simulink model "cb_pcidda_test"  (Simulink 4.00)
settings: Solver=FixedStepDiscrete  SolverMode=MultiTasking  StartTime=0.0  StopTime=1  RelTol=1e-3
libraries: cb_pcidda x7
CloseFcn:
  | rtwprivate ssgensfun ModelCloseRequest cb_pcidda_test
settings Model: Creator=dozio  LastModifiedBy=root  SimulationMode=external  RTWSystemTargetFile=grt_rtai.tlc  RTWOptions="-aBasePriority=30 -aExtMode=1 -aForceParamTrailComments=0 -aInlineInvariantSignals=0 -aInlineParameters=0 -aLocalBlockOutputs=1 -aLogVarNameModifier=\"rt_\" -aMatFileLogging=0 -aRTWVerbose=1 -aRollThreshold=5 -aShowEliminatedStatements=1 -aTaskStackSize=16384"  RTWTemplateMakefile=grt_rtai.tmf  BlockReductionOpt=off

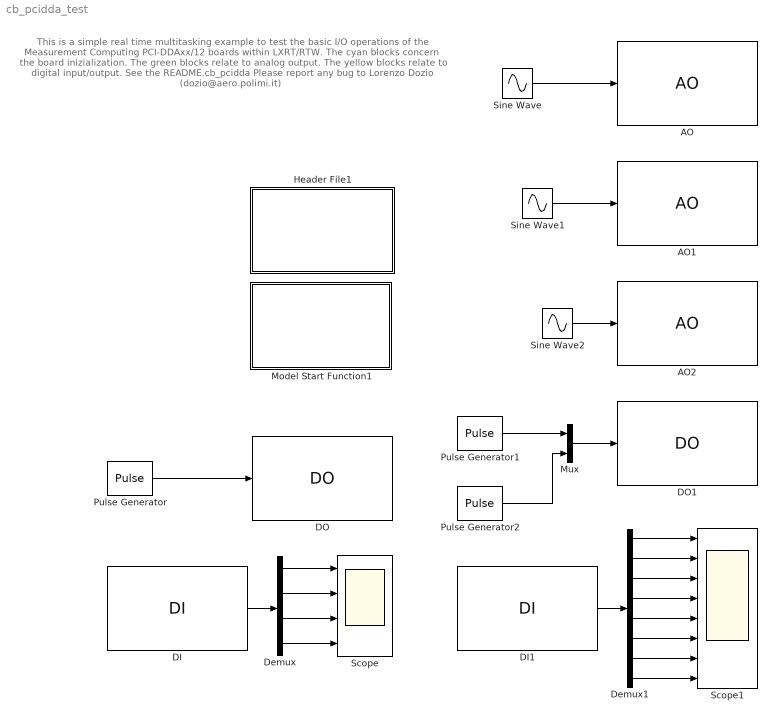
== system cb_pcidda_test ==
  note: This is a simple real time multitasking example to test
      | the basic I/O operations of the Measurement Computing
      | PCI-DDAxx/12 boards within LXRT/RTW.
      | The cyan blocks concern the board inizialization.
      | The green blocks relate to analog output.
      | The yellow blocks relate to digital input/output.
      | See the README.cb_pcidda
      |
      | Please report any bug to Lorenzo Dozio
      | (dozio@aero.polimi.it)
  AO : cb_pcidda/AO  chan=DAC0  pol=bipolar  vfs=10 V  dt=0.0001
  AO1 : cb_pcidda/AO  chan=DAC1  pol=unipolar  vfs=5 V  dt=0.0002
  AO2 : cb_pcidda/AO  chan=DAC2  pol=bipolar  vfs=10 V  dt=0.0004
  DI : cb_pcidda/DI  number=0  port=C_up  nchan=4  dt=0.0005
  DI1 : cb_pcidda/DI  number=1  port=A  nchan=8  dt=0.0005
  DO : cb_pcidda/DO  number=0  port=C_low  nchan=1  threshold=1  dt=0.0005
  DO1 : cb_pcidda/DO  number=1  port=B  nchan=2  threshold=1  dt=0.0005
  Demux : Demux  Outputs=4  BusSelectionMode=off
  Demux1 : Demux  Outputs=8  BusSelectionMode=off
  Header File1 : Subsystem  Tag=line1 line2
      settings: CopyFcn=cccopyfcn(gcb)  OpenFcn=ccopenfcn('Header File')  RTWFcnNameOpts=Auto  RTWFileNameOpts=Auto
      mask Type: Header File
      mask Description: Add code to model .h file
      mask Help: This header file block contains text fields to insert custom user code at the top and bottom of model.h file.
      mask Display: disp('Measurement Computing\nPCI-DDAxx/12\n\nHeader Files');
  Model Start Function1 : Subsystem
      settings: CopyFcn=cccopyfcn(gcb)  OpenFcn=ccopenfcn('Model Start Function')  RTWFcnNameOpts=Auto  RTWFileNameOpts=Auto
      mask Type: Model Start Function
      mask Description: Add code to Model Start function
      mask Help: This block contains text fields to insert custom user code sections at the declarations, execution and exit sections of the model start function.
      mask Display: disp('Measurement Computing\nPCI-DDAxx/12\n\nReset Digital I/O');
  Mux : Mux  Inputs=2
  Pulse Generator : DiscretePulseGenerator  Amplitude=2  Period=50  PulseWidth=25  PhaseDelay=0  SampleTime=0.0005
  Pulse Generator1 : DiscretePulseGenerator  Amplitude=2  Period=50  PulseWidth=25  PhaseDelay=0  SampleTime=0.0005
  Pulse Generator2 : DiscretePulseGenerator  Amplitude=2  Period=50  PulseWidth=25  PhaseDelay=0  SampleTime=0.0005
  Scope : Scope  NumInputPorts=4
      settings: TimeRange=0.1  YMin=0~0~0~0  YMax=1~1~1~1  SaveToWorkspace=off  LimitDataPoints=on  MaxDataPoints=5000
  Scope1 : Scope  NumInputPorts=8
      settings: TimeRange=0.1  YMin=0~0~0~0~0~0~0~0  YMax=1~1~1~1~1~1~1~1  SaveToWorkspace=off  SaveName=ScopeData  LimitDataPoints=on  MaxDataPoints=5000
  Sine Wave : Sin  Amplitude=5  Frequency=2*pi*50  Phase=0  SampleTime=0.0001
  Sine Wave1 : Sin  Amplitude=2.5  Frequency=2*pi*10  Phase=0  SampleTime=0.0002
  Sine Wave2 : Sin  Amplitude=2  Frequency=2*pi*50  Phase=0  SampleTime=0.0004
  wires:
  Sine Wave/1 -> AO/1
  Sine Wave1/1 -> AO1/1
  Sine Wave2/1 -> AO2/1
  Pulse Generator/1 -> DO/1
  DI/1 -> Demux/1
  Demux/1 -> Scope/1
  Demux/2 -> Scope/2
  Demux/3 -> Scope/3
  Demux/4 -> Scope/4
  Pulse Generator1/1 -> Mux/1
  Pulse Generator2/1 -> Mux/2
  Mux/1 -> DO1/1
  DI1/1 -> Demux1/1
  Demux1/1 -> Scope1/1
  Demux1/2 -> Scope1/2
  Demux1/4 -> Scope1/4
  Demux1/3 -> Scope1/3
  Demux1/5 -> Scope1/5
  Demux1/6 -> Scope1/6
  Demux1/7 -> Scope1/7
  Demux1/8 -> Scope1/8

== system cb_pcidda_test/Header File1 ==

== system cb_pcidda_test/Model Start Function1 ==
